simulink model "Integrated_ACC_LKS"  (Simulink 10.2)
settings: Solver=ode4  StartTime=0.0  StopTime=30  FixedStep=0.005  RelTol=1e-3  EnableMultiTasking=on
undefined symbols (not defined in the file or in its folder): sigbuilder_block
libraries: simulink x2
settings Model: Creator=Infineon02  LastModifiedBy=user
settings DataIOCC: SignalLoggingName=sigsOut
settings OptimizationCC: ExpressionDepthLimit=2147483647  InitFltsAndDblsToZero=on
settings DebuggingCC: SaveWithParameterizedLinksMsg=none  SignalResolutionControl=TryResolveAllWithWarning  MultiTaskDSMMsg=warning  MultiTaskCondExecSysMsg=none  StateNameClashWarn=warning
settings HardwareCC: TargetUnknown=on
settings GRTTargetCC: TargetFcnLib=ansi_tfl_tmw.mat

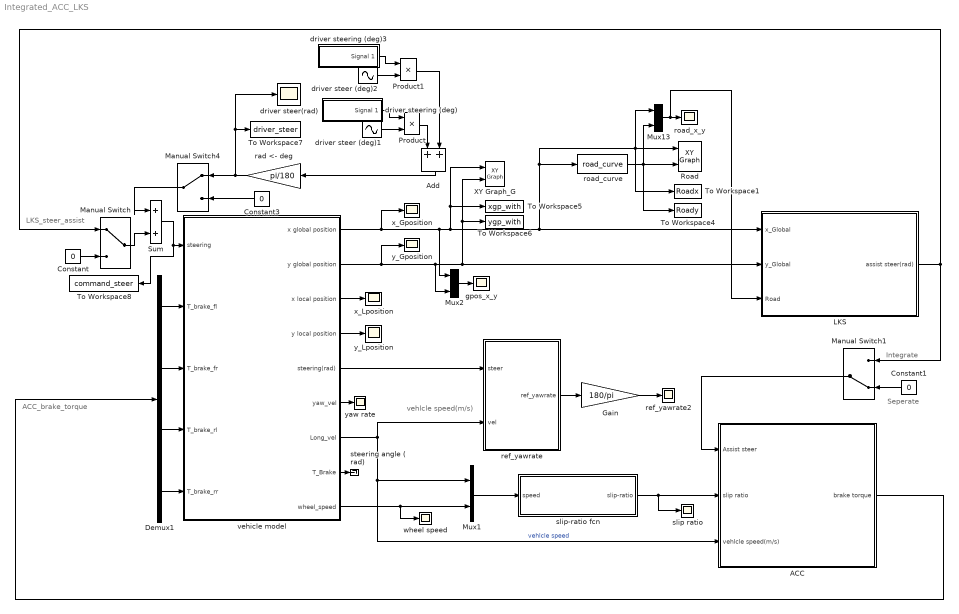
== system Integrated_ACC_LKS ==
  note: vehlcle speed(m/s)
  note: LKS_steer_assist
  note: ACC_brake_torque
  note: Seperate
  note: Integrate
  ACC : Subsystem
  Add : Sum
  Constant : Constant  Value=0
  Constant1 : Constant  Value=0
  Constant3 : Constant  Value=0
  Demux1 : Demux
      settings: DisplayOption=none
  Gain : Gain  Gain=180/pi  SaturateOnIntegerOverflow=on  OutDataTypeStr=Inherit: Same as input  ParamDataTypeStr=Inherit: Same as input
  LKS : Subsystem
  Manual Switch : ManualSwitch
  Manual Switch1 : ManualSwitch  CurrentSetting=0
  Manual Switch4 : ManualSwitch
  Mux1 : Mux  Inputs=2
  Mux13 : Mux  Inputs=2
  Mux2 : Mux  Inputs=2
  Product : Product  RndMeth=Zero
  Product1 : Product  RndMeth=Zero
  Road : simulink/Sinks/XY Graph  xmin=0  xmax=500  ymin=-100  ymax=1  st=0
  Sum : Sum  Inputs=|++  SaturateOnIntegerOverflow=on
  To Workspace1 : ToWorkspace  VariableName=Roadx  SampleTime=-1
  To Workspace4 : ToWorkspace  VariableName=Roady  SampleTime=-1
  To Workspace5 : ToWorkspace  VariableName=xgp_with  SampleTime=-1
  To Workspace6 : ToWorkspace  VariableName=ygp_with  SampleTime=-1
  To Workspace7 : ToWorkspace  VariableName=driver_steer  SampleTime=-1
  To Workspace8 : ToWorkspace  VariableName=command_steer  SampleTime=-1
  XY Graph_G : simulink/Sinks/XY Graph  xmin=0  xmax=500  ymin=-100  ymax=1  st=0
  driver steer (deg)1 : Sin  Amplitude=0.8  Frequency=0.34907  Phase=0.34898  SampleTime=0
  driver steer (deg)2 : Sin  Amplitude=0.8  Frequency=0.165347  Phase=2.64  SampleTime=0
  driver steer(rad) : Scope
  driver steering (deg) : Subsystem  Tag=STV Subsys  LoadFcn=sigbuilder_block('load');  StartFcn=sigbuilder_block('start');  StopFcn=sigbuilder_block('stop');  ClipboardFcn=sigbuilder_block('clipboard');  mask(Sigbuilder block){tuvar=[0:10]}
      mask help: Sigbuilder GUI
      mask init:
      | if ~strcmp(get_param(bdroot(gcbh),'SimulationStatus'),'stopped') tuvar = sigbuilder_block('maskInit'); end
      settings: CopyFcn=sigbuilder_block('copy');  DeleteFcn=sigbuilder_block('delete');  ModelCloseFcn=sigbuilder_block('modelClose');  PreSaveFcn=sigbuilder_block('preSave');  PauseFcn=sigbuilder_block('pause')  ContinueFcn=sigbuilder_block('continue')  NameChangeFcn=sigbuilder_block('namechange');  OpenFcn=sigbuilder_block('open',[323.25 135.75 558.75 274.5 ]);  CloseFcn=sigbuilder_block('close');
      mask Display: plot(0, 0, 100, 100,[2, 2, 32, 32, 2], [68, 8, 8, 68, 68],[32, 2], [38, 38], [32, 19, 2],[53, 60, 44], [32, 17, 17, 2],[16, 16, 31, 31]);txt = getActiveGroup(gcbh);text(2, 100, txt,'verticalAlignment', 'top');
  driver steering (deg)3 : Subsystem  Tag=STV Subsys  LoadFcn=sigbuilder_block('load');  StartFcn=sigbuilder_block('start');  StopFcn=sigbuilder_block('stop');  ClipboardFcn=sigbuilder_block('clipboard');  mask(Sigbuilder block){tuvar=[0:10]}
      mask help: Sigbuilder GUI
      mask init:
      | if ~strcmp(get_param(bdroot(gcbh),'SimulationStatus'),'stopped') tuvar = sigbuilder_block('maskInit'); end
      settings: CopyFcn=sigbuilder_block('copy');  DeleteFcn=sigbuilder_block('delete');  ModelCloseFcn=sigbuilder_block('modelClose');  PreSaveFcn=sigbuilder_block('preSave');  PauseFcn=sigbuilder_block('pause')  ContinueFcn=sigbuilder_block('continue')  NameChangeFcn=sigbuilder_block('namechange');  OpenFcn=sigbuilder_block('open',[323.25 135.75 558.75 274.5 ]);  CloseFcn=sigbuilder_block('close');
      mask Display: plot(0, 0, 100, 100,[2, 2, 32, 32, 2], [68, 8, 8, 68, 68],[32, 2], [38, 38], [32, 19, 2],[53, 60, 44], [32, 17, 17, 2],[16, 16, 31, 31]);txt = getActiveGroup(gcbh);text(2, 100, txt,'verticalAlignment', 'top');
  gpos_x_y : Scope
  rad <- deg : Gain  Gain=pi/180  SaturateOnIntegerOverflow=on  OutDataTypeStr=Inherit: Same as input  ParamDataTypeStr=Inherit: Same as input
  ref_yawrate : Subsystem
  ref_yawrate2 : Scope
  road_curve : MATLABFcn  MATLABFcn=road_curve
  road_x_y : Scope
  slip ratio : Scope
  slip-ratio fcn : Subsystem
  steering angle ( rad) : Terminator
  vehicle model : Subsystem
  wheel speed : Scope
  x_Gposition : Scope
  x_Lposition : Scope
  y_Gposition : Scope
  y_Lposition : Scope
  yaw rate : Scope
  wires:
  vehicle model/7(Long_vel) -> ref_yawrate/2(vel), Mux1/1, ACC/3(vehlcle speed(m/s))  "vehlcle speed"
  ref_yawrate/1(ref_yawrate) -> Gain/1
  vehicle model/6(yaw_vel) -> yaw rate/1
  Mux1/1 -> slip-ratio fcn/1(speed)
  vehicle model/9(wheel_speed) -> Mux1/2, wheel speed/1
  Constant/1 -> Manual Switch/2
  Gain/1 -> ref_yawrate2/1
  vehicle model/3(x local position) -> x_Lposition/1
  vehicle model/8(T_Brake) -> steering angle ( rad)/1
  vehicle model/4(y local position) -> y_Lposition/1
  driver steer (deg)1/1 -> Product/2
  driver steering (deg)/1(Signal 1) -> Product/1
  Mux13/1 -> road_x_y/1, LKS/3(Road)
  road_curve/1 -> Mux13/2, Road/2, To Workspace4/1
  Manual Switch/1 -> Sum/2
  Sum/1 -> vehicle model/1(steering), To Workspace8/1
  vehicle model/5(steering(rad)) -> ref_yawrate/1(steer)
  vehicle model/1(x global position) -> x_Gposition/1, Mux13/1, Road/1, To Workspace1/1, road_curve/1, LKS/1(x_Global), To Workspace5/1, XY Graph_G/1, Mux2/1
  rad <- deg/1 -> Manual Switch4/1, driver steer(rad)/1, To Workspace7/1
  Manual Switch4/1 -> Sum/1
  Constant3/1 -> Manual Switch4/2
  Demux1/4 -> vehicle model/5(T_brake_rr)
  Demux1/3 -> vehicle model/4(T_brake_rl)
  Demux1/2 -> vehicle model/3(T_brake_fr)
  Demux1/1 -> vehicle model/2(T_brake_fl)
  vehicle model/2(y global position) -> y_Gposition/1, To Workspace6/1, XY Graph_G/2, LKS/2(y_Global), Mux2/2
  LKS/1(assist steer(rad)) -> Manual Switch/1, Manual Switch1/1
  ACC/1(brake torque) -> Demux1/1
  Add/1 -> rad <- deg/1
  slip-ratio fcn/1(slip-ratio) -> ACC/2(slip ratio), slip ratio/1
  Manual Switch1/1 -> ACC/1(Assist steer)
  Constant1/1 -> Manual Switch1/2
  driver steer (deg)2/1 -> Product1/2
  driver steering (deg)3/1(Signal 1) -> Product1/1
  Product/1 -> Add/1
  Product1/1 -> Add/2
  Mux2/1 -> gpos_x_y/1

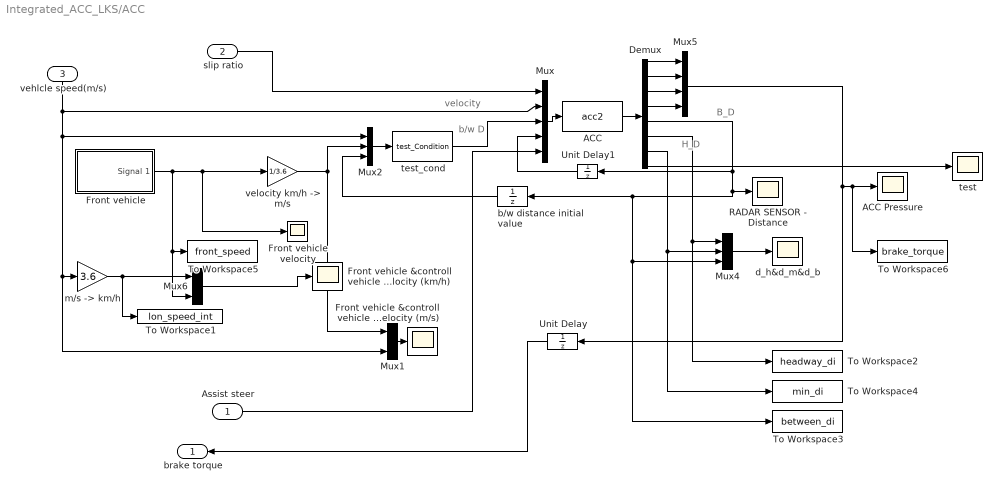
== system Integrated_ACC_LKS/ACC ==
  note: velocity
  note: H_D
  note: B_D
  note: b/w D
  Assist steer : Inport
  slip ratio : Inport  Port=2
  vehlcle speed(m/s) : Inport  Port=3
  ACC : MATLABFcn  MATLABFcn=acc2
  ACC Pressure : Scope
  Demux : Demux  Outputs=8
  Front vehicle : Subsystem  Tag=STV Subsys  LoadFcn=sigbuilder_block('load');  StartFcn=sigbuilder_block('start');  StopFcn=sigbuilder_block('stop');  ClipboardFcn=sigbuilder_block('clipboard');  mask(Sigbuilder block){tuvar=[0:10]}
      mask help: Sigbuilder GUI
      mask init:
      | if ~strcmp(get_param(bdroot(gcbh),'SimulationStatus'),'stopped') tuvar = sigbuilder_block('maskInit'); end
      settings: CopyFcn=sigbuilder_block('copy');  DeleteFcn=sigbuilder_block('delete');  ModelCloseFcn=sigbuilder_block('modelClose');  PreSaveFcn=sigbuilder_block('preSave');  PauseFcn=sigbuilder_block('pause')  ContinueFcn=sigbuilder_block('continue')  NameChangeFcn=sigbuilder_block('namechange');  OpenFcn=sigbuilder_block('open',[306.75 214.5 550.5 399.75 ]);  CloseFcn=sigbuilder_block('close');
      mask Display: plot(0, 0, 100, 100,[2, 2, 32, 32, 2], [68, 8, 8, 68, 68],[32, 2], [38, 38], [32, 19, 2],[53, 60, 44], [32, 17, 17, 2],[16, 16, 31, 31]);txt = getActiveGroup(gcbh);text(2, 100, txt,'verticalAlignment', 'top');
  Front vehicle &controll vehicle velocity (km/h) : Scope
  Front vehicle &controll vehicle velocity (m/s) : Scope
  Front vehicle velocity : Scope
  Mux : Mux  Inputs=5
  Mux1 : Mux  Inputs=2
  Mux2 : Mux  Inputs=3
  Mux4 : Mux  Inputs=3
  Mux5 : Mux
  Mux6 : Mux  Inputs=2
  RADAR SENSOR - Distance : Scope
  To Workspace1 : ToWorkspace  VariableName=lon_speed_int  SampleTime=-1
  To Workspace2 : ToWorkspace  VariableName=headway_di  SampleTime=-1
  To Workspace3 : ToWorkspace  VariableName=between_di  SampleTime=-1
  To Workspace4 : ToWorkspace  VariableName=min_di  SampleTime=-1
  To Workspace5 : ToWorkspace  VariableName=front_speed  SampleTime=-1
  To Workspace6 : ToWorkspace  VariableName=brake_torque  SampleTime=-1
  Unit Delay : UnitDelay  SampleTime=0.005  HasFrameUpgradeWarning=on
  Unit Delay1 : UnitDelay  InitialCondition=55  SampleTime=-1  HasFrameUpgradeWarning=on
  b/w distance initial value : UnitDelay  InitialCondition=55  SampleTime=-1  HasFrameUpgradeWarning=on
  d_h&d_m&d_b : Scope
  "m/s -> km/h" : Gain  Gain=3.6
  test : Scope
  test_cond : MATLABFcn  MATLABFcn=test_Condition
  "velocity km/h -> m/s" : Gain  Gain=1/3.6  SaturateOnIntegerOverflow=on  OutDataTypeStr=Inherit: Same as input  ParamDataTypeStr=Inherit: Same as input
  brake torque : Outport
  wires:
  ACC/1 -> Demux/1
  Mux2/1 -> test_cond/1
  Demux/1 -> Mux5/1
  Demux/2 -> Mux5/2
  Demux/3 -> Mux5/3
  Demux/4 -> Mux5/4
  Demux/5 -> RADAR SENSOR - Distance/1, b/w distance initial value/1, To Workspace3/1, Mux4/3, Unit Delay1/1
  test_cond/1 -> Mux/3
  b/w distance initial value/1 -> Mux2/3
  Front vehicle/1(Signal 1) -> "velocity km/h -> m/s"/1, Front vehicle velocity/1, Mux6/2, To Workspace5/1
  "velocity km/h -> m/s"/1 -> Mux2/2, Mux1/1
  Demux/6 -> Mux4/1, To Workspace2/1
  Mux5/1 -> Unit Delay/1, ACC Pressure/1, To Workspace6/1
  Unit Delay1/1 -> Mux/4
  Mux6/1 -> Front vehicle &controll vehicle velocity (km/h)/1
  Mux4/1 -> d_h&d_m&d_b/1
  Mux/1 -> ACC/1
  "m/s -> km/h"/1 -> Mux6/1, To Workspace1/1
  vehlcle speed(m/s)/1 -> Mux/2, Mux2/1, "m/s -> km/h"/1, Mux1/2
  slip ratio/1 -> Mux/1
  Unit Delay/1 -> brake torque/1
  Assist steer/1 -> Mux/5
  Demux/7 -> Mux4/2, To Workspace4/1
  Demux/8 -> test/1
  Mux1/1 -> Front vehicle &controll vehicle velocity (m/s)/1

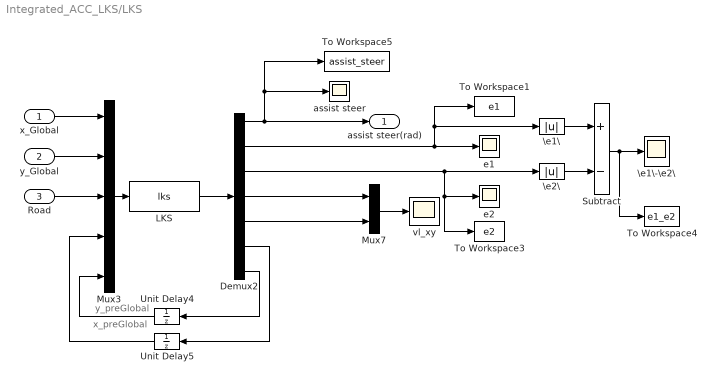
== system Integrated_ACC_LKS/LKS ==
  note: x_preGlobal
  note: y_preGlobal
  x_Global : Inport
  y_Global : Inport  Port=2
  Road : Inport  Port=3
  Demux2 : Demux  Outputs=7
  LKS : MATLABFcn  MATLABFcn=lks
  Mux3 : Mux  Inputs=5
  Mux7 : Mux  Inputs=2
  Subtract : Sum  Inputs=+-
  To Workspace1 : ToWorkspace  VariableName=e1  SampleTime=-1
  To Workspace3 : ToWorkspace  VariableName=e2  SampleTime=-1
  To Workspace4 : ToWorkspace  VariableName=e1_e2  SampleTime=-1
  To Workspace5 : ToWorkspace  VariableName=assist_steer  SampleTime=-1
  Unit Delay4 : UnitDelay  SampleTime=-1  HasFrameUpgradeWarning=on
  Unit Delay5 : UnitDelay  SampleTime=-1  HasFrameUpgradeWarning=on
  \e1\ : Abs
  \e1\-\e2\ : Scope
  \e2\ : Abs
  assist steer : Scope
  e1 : Scope
  e2 : Scope
  vl_xy : Scope
  assist steer(rad) : Outport
  wires:
  Demux2/7 -> Unit Delay4/1
  Unit Delay4/1 -> Mux3/5
  Demux2/6 -> Unit Delay5/1
  Unit Delay5/1 -> Mux3/4
  Demux2/5 -> Mux7/2
  Demux2/4 -> Mux7/1
  Demux2/3 -> \e2\/1, e2/1, To Workspace3/1
  Mux7/1 -> vl_xy/1
  Demux2/2 -> e1/1, \e1\/1, To Workspace1/1
  Demux2/1 -> assist steer(rad)/1, assist steer/1, To Workspace5/1
  LKS/1 -> Demux2/1
  Mux3/1 -> LKS/1
  x_Global/1 -> Mux3/1
  y_Global/1 -> Mux3/2
  Road/1 -> Mux3/3
  \e1\/1 -> Subtract/1
  \e2\/1 -> Subtract/2
  Subtract/1 -> \e1\-\e2\/1, To Workspace4/1

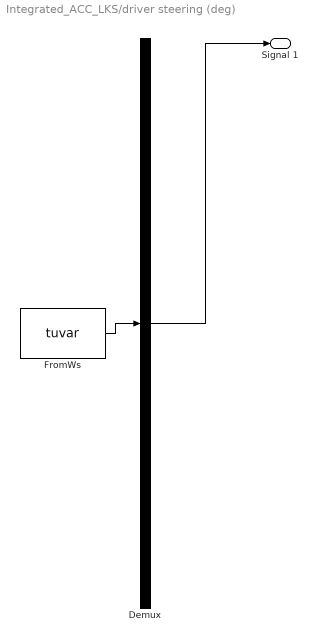
== system Integrated_ACC_LKS/driver steering (deg) ==
  Demux : Demux  Tag=STV Demux  Outputs=1
      settings: DisplayOption=none
  FromWs : FromWorkspace  Tag=STV FromWs  VariableName=tuvar  SigBuilderData=DataTag2  VnvData=DataTag3
      SigBuilderData=|
      | common.afterFinalStr = 'Extrapolate'
      | common.sampleTime = 0
      | dataSet.timeRange = [0 30]
      | dataSet.name = 'Group 1'
      | sbobj.Groups.Name = 'Group 1'
      | sbobj.Groups.Signals.Name = 'Signal 1'
      | sbobj.Groups.Signals.XData = [0 8 8 12.6 12.6 30]
      | sbobj.Groups.Signals.YData = [0 0 1 1 0 0]
      | sbobj.Groups.TimeRange = [0 30]
  Signal 1 : Outport  Tag=STV Outport
  wires:
  FromWs/1 -> Demux/1
  Demux/1 -> Signal 1/1

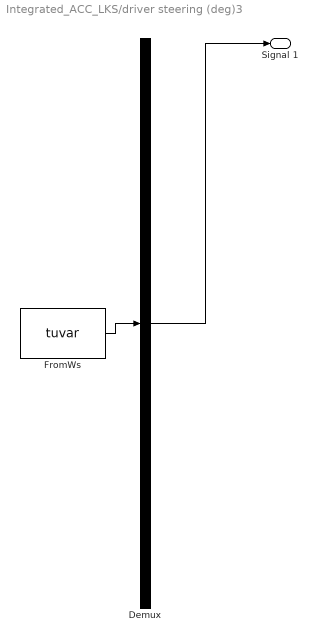
== system Integrated_ACC_LKS/driver steering (deg)3 ==
  Demux : Demux  Tag=STV Demux  Outputs=1
      settings: DisplayOption=none
  FromWs : FromWorkspace  Tag=STV FromWs  VariableName=tuvar  SigBuilderData=DataTag4  VnvData=DataTag5
      SigBuilderData=|
      | common.afterFinalStr = 'Extrapolate'
      | common.sampleTime = 0
      | dataSet.timeRange = [0 30]
      | dataSet.name = 'Group 1'
      | sbobj.Groups.Name = 'Group 1'
      | sbobj.Groups.Signals.Name = 'Signal 1'
      | sbobj.Groups.Signals.XData = [0 12.6 12.6 22 22 30]
      | sbobj.Groups.Signals.YData = [0 0 1 1 0 0]
      | sbobj.Groups.TimeRange = [0 30]
  Signal 1 : Outport  Tag=STV Outport
  wires:
  Demux/1 -> Signal 1/1
  FromWs/1 -> Demux/1

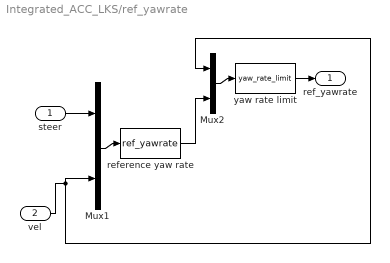
== system Integrated_ACC_LKS/ref_yawrate ==
  steer : Inport
  vel : Inport  Port=2
  Mux1 : Mux  Inputs=2
  Mux2 : Mux  Inputs=2
  reference yaw rate : MATLABFcn  MATLABFcn=ref_yawrate
  yaw rate limit : MATLABFcn  MATLABFcn=yaw_rate_limit
  ref_yawrate : Outport
  wires:
  Mux1/1 -> reference yaw rate/1
  reference yaw rate/1 -> Mux2/2
  Mux2/1 -> yaw rate limit/1
  vel/1 -> Mux1/2, Mux2/1
  yaw rate limit/1 -> ref_yawrate/1
  steer/1 -> Mux1/1

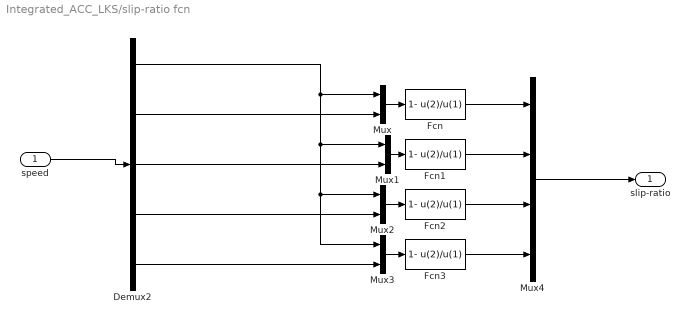
== system Integrated_ACC_LKS/slip-ratio fcn ==
  speed : Inport
  Demux2 : Demux  Outputs=5
      settings: DisplayOption=none
  Fcn{,1..3} (4 alike) : Fcn  Expr=1- u(2)/u(1)
  Mux{,1..3} (4 alike) : Mux  Inputs=2
  Mux4 : Mux
  slip-ratio : Outport
  wires:
  Mux/1 -> Fcn/1
  Demux2/1 -> Mux/1, Mux1/1, Mux2/1, Mux3/1
  Mux1/1 -> Fcn1/1
  Mux2/1 -> Fcn2/1
  Mux3/1 -> Fcn3/1
  Fcn/1 -> Mux4/1
  Fcn1/1 -> Mux4/2
  Fcn2/1 -> Mux4/3
  Fcn3/1 -> Mux4/4
  Mux4/1 -> slip-ratio/1
  Demux2/2 -> Mux/2
  Demux2/3 -> Mux1/2
  Demux2/4 -> Mux2/2
  Demux2/5 -> Mux3/2
  speed/1 -> Demux2/1

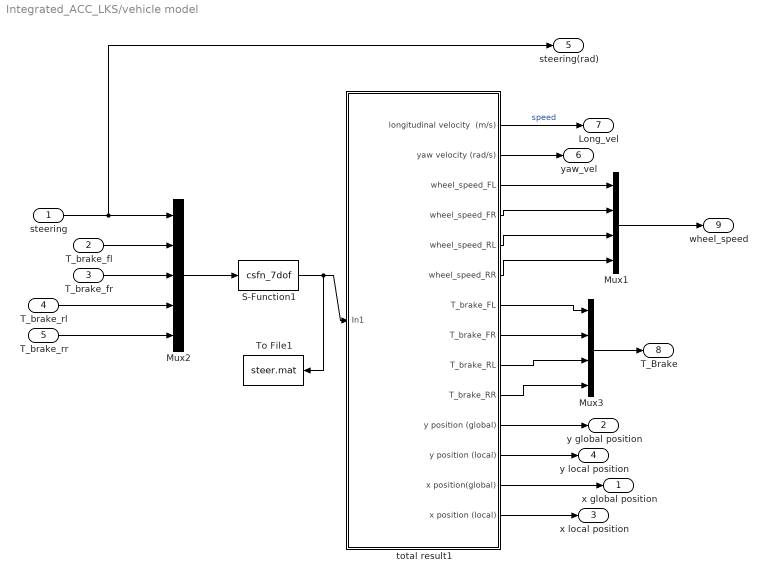
== system Integrated_ACC_LKS/vehicle model ==
  steering : Inport
  T_brake_fl : Inport  Port=2
  T_brake_fr : Inport  Port=3
  T_brake_rl : Inport  Port=4
  T_brake_rr : Inport  Port=5
  Mux1 : Mux
  Mux2 : Mux  Inputs=5
  Mux3 : Mux
  S-Function1 : S-Function  FunctionName=csfn_7dof  SFunctionDeploymentMode=off  EnableBusSupport=off
  To File1 : ToFile  Filename=steer.mat  MatrixName=steer
  total result1 : Subsystem
  x global position : Outport
  y global position : Outport  Port=2
  x local position : Outport  Port=3
  y local position : Outport  Port=4
  steering(rad) : Outport  Port=5
  yaw_vel : Outport  Port=6
  Long_vel : Outport  Port=7
  T_Brake : Outport  Port=8
  wheel_speed : Outport  Port=9
  wires:
  S-Function1/1 -> total result1/1(In1), To File1/1
  total result1/1(longitudinal velocity  (m/s)) -> Long_vel/1  "speed"
  steering/1 -> Mux2/1, steering(rad)/1
  Mux2/1 -> S-Function1/1
  T_brake_fl/1 -> Mux2/2
  T_brake_fr/1 -> Mux2/3
  T_brake_rl/1 -> Mux2/4
  T_brake_rr/1 -> Mux2/5
  total result1/2(yaw velocity (rad/s)) -> yaw_vel/1
  total result1/3(wheel_speed_FL) -> Mux1/1
  total result1/4(wheel_speed_FR) -> Mux1/2
  total result1/5(wheel_speed_RL) -> Mux1/3
  total result1/6(wheel_speed_RR) -> Mux1/4
  total result1/7(T_brake_FL) -> Mux3/1
  total result1/8(T_brake_FR) -> Mux3/2
  total result1/9(T_brake_RL) -> Mux3/3
  total result1/10(T_brake_RR) -> Mux3/4
  Mux3/1 -> T_Brake/1
  total result1/11(y position (global)) -> y global position/1
  total result1/12(y position (local)) -> y local position/1
  total result1/13(x position(global)) -> x global position/1
  total result1/14(x position (local)) -> x local position/1
  Mux1/1 -> wheel_speed/1

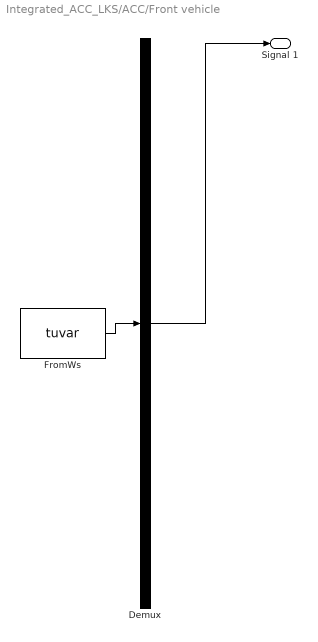
== system Integrated_ACC_LKS/ACC/Front vehicle ==
  Demux : Demux  Tag=STV Demux  Outputs=1
      settings: DisplayOption=none
  FromWs : FromWorkspace  Tag=STV FromWs  VariableName=tuvar  SigBuilderData=DataTag0  VnvData=DataTag1
      SigBuilderData=|
      | common.afterFinalStr = 'Extrapolate'
      | common.sampleTime = 0
      | dataSet.timeRange = [0 30]
      | dataSet.name = 'Group 1'
      | sbobj.Groups.Name = 'Group 1'
      | sbobj.Groups.Signals.Name = 'Signal 1'
      | sbobj.Groups.Signals.XData = [0 10 20 25 30]
      | sbobj.Groups.Signals.YData = [70 70 25.5 25.5 25.5]
      | sbobj.Groups.TimeRange = [0 30]
  Signal 1 : Outport  Tag=STV Outport
  wires:
  Demux/1 -> Signal 1/1
  FromWs/1 -> Demux/1

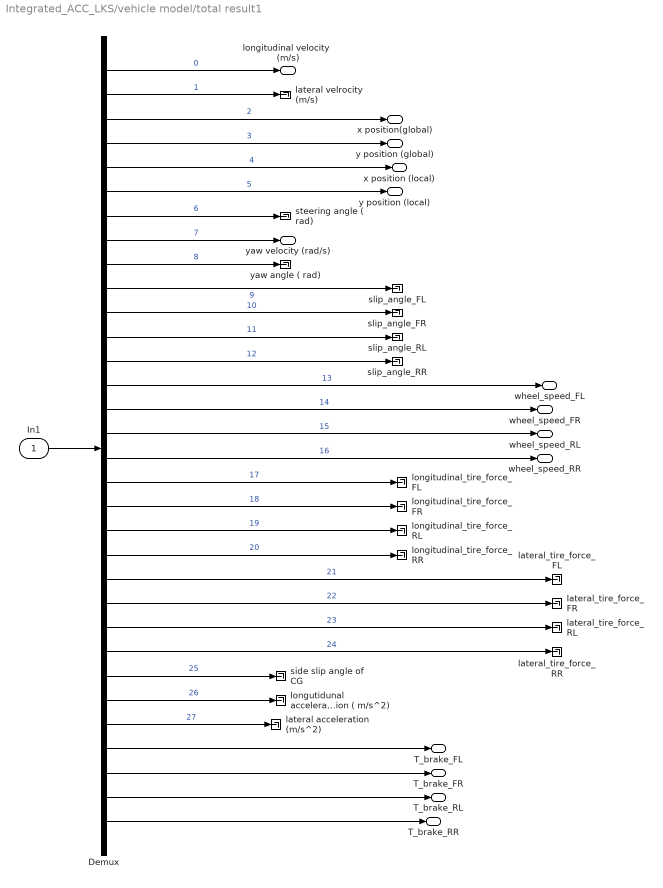
== system Integrated_ACC_LKS/vehicle model/total result1 ==
  In1 : Inport
  Demux : Demux  Outputs=32
      settings: DisplayOption=none
  lateral acceleration (m/s^2) : Terminator
  lateral velrocity (m/s) : Terminator
  lateral_tire_force_FL : Terminator
  lateral_tire_force_FR : Terminator
  lateral_tire_force_RL : Terminator
  lateral_tire_force_RR : Terminator
  longitudinal_tire_force_FL : Terminator
  longitudinal_tire_force_FR : Terminator
  longitudinal_tire_force_RL : Terminator
  longitudinal_tire_force_RR : Terminator
  longutidunal acceleration ( m/s^2) : Terminator
  side slip angle of CG : Terminator
  slip_angle_FL : Terminator
  slip_angle_FR : Terminator
  slip_angle_RL : Terminator
  slip_angle_RR : Terminator
  steering angle ( rad) : Terminator
  yaw angle ( rad) : Terminator
  longitudinal velocity  (m/s) : Outport
  yaw velocity (rad/s) : Outport  Port=2
  wheel_speed_FL : Outport  Port=3
  wheel_speed_FR : Outport  Port=4
  wheel_speed_RL : Outport  Port=5
  wheel_speed_RR : Outport  Port=6
  T_brake_FL : Outport  Port=7
  T_brake_FR : Outport  Port=8
  T_brake_RL : Outport  Port=9
  T_brake_RR : Outport  Port=10
  y position (global) : Outport  Port=11
  y position (local) : Outport  Port=12
  x position(global) : Outport  Port=13
  x position (local) : Outport  Port=14
  wires:
  Demux/1 -> longitudinal velocity  (m/s)/1  "0"
  Demux/2 -> lateral velrocity (m/s)/1  "1"
  Demux/8 -> yaw velocity (rad/s)/1  "7"
  Demux/3 -> x position(global)/1  "2"
  Demux/14 -> wheel_speed_FL/1  "13"
  Demux/13 -> slip_angle_RR/1  "12"
  Demux/12 -> slip_angle_RL/1  "11"
  Demux/11 -> slip_angle_FR/1  "10"
  Demux/10 -> slip_angle_FL/1  "9"
  Demux/9 -> yaw angle ( rad)/1  "8"
  Demux/7 -> steering angle ( rad)/1  "6"
  Demux/6 -> y position (local)/1  "5"
  Demux/5 -> x position (local)/1  "4"
  Demux/4 -> y position (global)/1  "3"
  In1/1 -> Demux/1
  Demux/15 -> wheel_speed_FR/1  "14"
  Demux/16 -> wheel_speed_RL/1  "15"
  Demux/17 -> wheel_speed_RR/1  "16"
  Demux/18 -> longitudinal_tire_force_FL/1  "17"
  Demux/19 -> longitudinal_tire_force_FR/1  "18"
  Demux/20 -> longitudinal_tire_force_RL/1  "19"
  Demux/21 -> longitudinal_tire_force_RR/1  "20"
  Demux/22 -> lateral_tire_force_FL/1  "21"
  Demux/23 -> lateral_tire_force_FR/1  "22"
  Demux/24 -> lateral_tire_force_RL/1  "23"
  Demux/25 -> lateral_tire_force_RR/1  "24"
  Demux/26 -> side slip angle of CG/1  "25"
  Demux/27 -> longutidunal acceleration ( m/s^2)/1  "26"
  Demux/28 -> lateral acceleration (m/s^2)/1  "27"
  Demux/29 -> T_brake_FL/1
  Demux/30 -> T_brake_FR/1
  Demux/31 -> T_brake_RL/1
  Demux/32 -> T_brake_RR/1
